simulink subsystem "PSC_AccelPdl"  (R2023a)
settings: Solver=VariableStepAuto  StartTime=0.0  StopTime=10.0  RelTol=1e-3
undefined symbols (not defined in the file or in its folder): TqCmd_Final_Forward, TqCmd_Final_Reverse
undefined symbols (not defined in the file): CAN2, ETRS, Tx
libraries: simulink x2
settings Model: Creator=edward9  LastModifiedBy=tstic

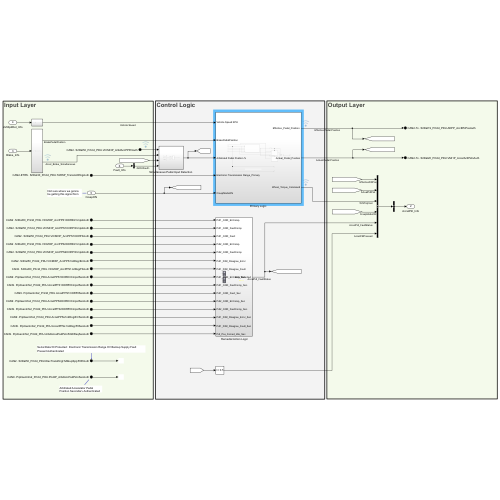
[thumbnail: Simulink's stored preview of the top-level diagram]
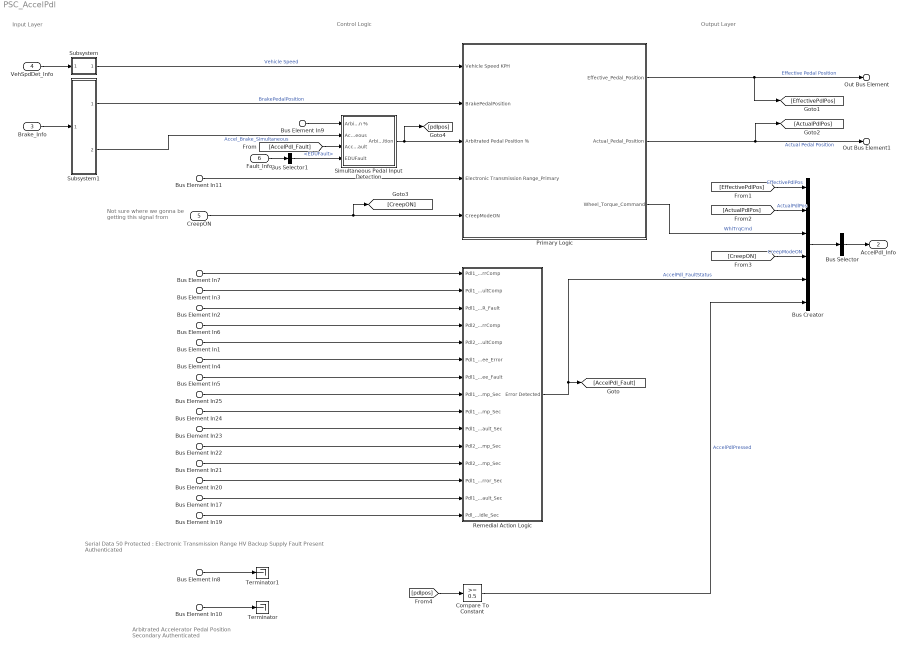
== system PSC_AccelPdl ==
  note: Output Layer
  note: Control Logic
  note: Input Layer
  note: Not sure where we gonna be getting this signal from
  note: Arbitrated Accelerator Pedal Position Secondary Authenticated
  note: Serial Data 50 Protected : Electronic Transmission Range HV Backup Supply Fault Present Authenticated
  Bus Element In7 : Inport  PortName=CAN2  Element=ID102_SrlDat50_Prtctd_PDU.VICMI3P_AccPPS1OORErrCmpstAuth
  Bus Element In3 : Inport  PortName=CAN2  Element=ID102_SrlDat50_Prtctd_PDU.VICMI3P_AccPPS1OORFltCmpstAuth
  Bus Element In2 : Inport  PortName=CAN2  Element=ID102_SrlDat50_Prtctd_PDU.VICMI3P_AccPPS1OORFltAuth
  Bus Element In6 : Inport  PortName=CAN2  Element=ID102_SrlDat50_Prtctd_PDU.VICMI3P_AccPPS2OORErrCmpstAuth
  Bus Element In1 : Inport  PortName=CAN2  Element=ID102_SrlDat50_Prtctd_PDU.VICMI3P_AccPPS2OORFltCmpstAuth
  Bus Element In4 : Inport  PortName=CAN2  Element=ID102_SrlDat50_Prtctd_PDU.VICMI3P_AccPPS1n2DsgrErrAuth
  Bus Element In5 : Inport  PortName=CAN2  Element=ID102_SrlDat50_Prtctd_PDU.VICMI3P_AccPPS1n2DsgrFltAuth
  Bus Element In8 : Inport  PortName=CAN2  Element=ID102_SrlDat50_Prtctd_PDU.ElecTransRngHVBkupSplyFltPrAuth
  Bus Element In9 : Inport  PortName=CAN2  Element=ID102_SrlDat50_Prtctd_PDU.VICMI3P_ArbdAccPPPriAuth
  Bus Element In10 : Inport  Port=2  PortName=CAN9  Element=ID106_PrplGenInfo2_Prtctd_PDU.PGI2P_ArbdAccPedPstnSecAuth
  Bus Element In25 : Inport  Port=2  PortName=CAN9  Element=ID106_PrplGenInfo2_Prtctd_PDU.AccelPPS1OORErrCmpstSecAuth
  Bus Element In24 : Inport  Port=2  PortName=CAN9  Element=ID106_PrplGenInfo2_Prtctd_PDU.AccelPPS1OORFltCmpstSecAuth
  Bus Element In23 : Inport  Port=2  PortName=CAN9  Element=ID106_PrplGenInfo2_Prtctd_PDU.AccelPPS1OORFltSecAuth
  Bus Element In22 : Inport  Port=2  PortName=CAN9  Element=ID106_PrplGenInfo2_Prtctd_PDU.AccelPPS2OORErrCmpstSecAuth
  Bus Element In21 : Inport  Port=2  PortName=CAN9  Element=ID106_PrplGenInfo2_Prtctd_PDU.AccelPPS2OORFltCmpstSecAuth
  Bus Element In20 : Inport  Port=2  PortName=CAN9  Element=ID106_PrplGenInfo2_Prtctd_PDU.AccelPPSs1n2DsgrErrSecAuth
  Bus Element In17 : Inport  Port=2  PortName=CAN9  Element=ID106_PrplGenInfo2_Prtctd_PDU.AccelPPSs1n2DsgrFltSecAuth
  Bus Element In19 : Inport  Port=2  PortName=CAN9  Element=ID106_PrplGenInfo2_Prtctd_PDU.ArbdAccelPedPstnFdIdlReqSecAuth
  Brake_Info : Inport  Port=3
  VehSpdDet_Info : Inport  Port=4
  CreepON : Inport  Port=5
  Fault_Info : Inport  Port=6
  Bus Element In11 : Inport  Port=7  PortName=CAN2-ETRS  Element=SrlDat30_Prtctd_PDU.TARSP_TransActlRngAuth
  " Remedial Action Logic" : Subsystem
  Bus Creator : BusCreator  Inputs=6
  Bus Selector : BusSelector  OutputSignals=EffectivePdlPos,ActualPdlPos,WhlTrqCmd,CreepModeON,AccelPdl_FaultStatus,AccelPdlPressed  OutputAsBus=on
  Bus Selector1 : BusSelector  OutputSignals=EDUFault
  Compare To Constant : simulink/Logic and Bit Operations/Compare To Constant  relop=>=  const=0.5  OutDataTypeStr=boolean
  "Primary Logic " : Subsystem
  "Simultaneous Pedal Input Detection " : Subsystem
  Subsystem : Subsystem
  Subsystem1 : Subsystem
  Terminator : Terminator
  Terminator1 : Terminator
  Out Bus Element : Outport  PortName=CAN2-Tx  Element=SrlDat19_Prtctd_PDU.AEPP_AccEffcPosAuth
  Out Bus Element1 : Outport  PortName=CAN2-Tx  Element=SrlDat20_Prtctd_PDU.VMI1P_AccelActlPstnAuth
  AccelPdl_Info : Outport  Port=2
  wires:
  Bus Element In11/1 -> "Primary Logic "/4(Electronic Transmission Range_Primary)
  " Remedial Action Logic"/1("Error Detected ") -> [AccelPdl_Fault], Bus Creator/5  "AccelPdl_FaultStatus"
  "Primary Logic "/3(Wheel_Torque_Command) -> Bus Creator/3  "WhlTrqCmd"
  "Primary Logic "/2(Actual_Pedal_Position) -> Out Bus Element1/1, [ActualPdlPos]  "Actual Pedal Position"
  "Primary Logic "/1("Effective_Pedal_Position ") -> Out Bus Element/1, [EffectivePdlPos]  "Effective Pedal Position"
  Bus Element In7/1 -> " Remedial Action Logic"/1(Pdl1_OOR_ErrComp)
  Bus Element In3/1 -> " Remedial Action Logic"/2(Pdl1_OOR_FaultComp)
  Bus Element In2/1 -> " Remedial Action Logic"/3(Pdl1_OOR_Fault)
  Bus Element In6/1 -> " Remedial Action Logic"/4(Pdl2_OOR_ErrComp)
  Bus Element In1/1 -> " Remedial Action Logic"/5(Pdl2_OOR_FaultComp)
  Bus Element In4/1 -> " Remedial Action Logic"/6(Pdl1_Pdl2_Disagree_Error)
  Bus Element In5/1 -> " Remedial Action Logic"/7(Pdl1_Pdl2_Disagree_Fault)
  "Simultaneous Pedal Input Detection "/1(Arbitrated Pedal Position) -> "Primary Logic "/3("Arbitrated Pedal Position % "), [pdlpos]
  Bus Element In25/1 -> " Remedial Action Logic"/8(Pdl1_OOR_ErrComp_Sec)
  Bus Element In24/1 -> " Remedial Action Logic"/9(Pdl1_OOR_FaultComp_Sec)
  Bus Element In23/1 -> " Remedial Action Logic"/10(Pdl1_OOR_Fault_Sec)
  Bus Element In22/1 -> " Remedial Action Logic"/11(Pdl2_OOR_ErrComp_Sec)
  Bus Element In21/1 -> " Remedial Action Logic"/12(Pdl2_OOR_FaultComp_Sec)
  Bus Element In20/1 -> " Remedial Action Logic"/13(Pdl1_Pdl2_Disagree_Error_Sec)
  Bus Element In17/1 -> " Remedial Action Logic"/14(Pdl1_Pdl2_Disagree_Fault_Sec)
  Bus Element In19/1 -> " Remedial Action Logic"/15(Pdl_Pos_Forced_Idle_Sec)
  CreepON/1 -> "Primary Logic "/5(CreepModeON), [CreepON]
  Bus Element In10/1 -> Terminator/1
  Bus Element In8/1 -> Terminator1/1
  VehSpdDet_Info/1 -> Subsystem/1(In1)
  Subsystem/1(VehSpd) -> "Primary Logic "/1(Vehicle Speed KPH)  "Vehicle Speed"
  Brake_Info/1 -> Subsystem1/1(Brake_Info)
  Subsystem1/1(BrakePedalPosition) -> "Primary Logic "/2(BrakePedalPosition)  "BrakePedalPosition"
  Subsystem1/2(Accel_Brake_Simultaneous) -> "Simultaneous Pedal Input Detection "/2(Accel_Brake_Simultaneous)  "Accel_Brake_Simultaneous"
  Bus Element In9/1 -> "Simultaneous Pedal Input Detection "/1("Arbitrated Pedal Position % ")
  Bus Creator/1 -> Bus Selector/1
  Bus Selector/1 -> AccelPdl_Info/1
  [AccelPdl_Fault] -> "Simultaneous Pedal Input Detection "/3(AccelPdl_Fault)
  [EffectivePdlPos] -> Bus Creator/1  "EffectivePdlPos"
  [ActualPdlPos] -> Bus Creator/2  "ActualPdlPos"
  [CreepON] -> Bus Creator/4  "CreepModeON"
  [pdlpos] -> Compare To Constant/1
  Compare To Constant/1 -> Bus Creator/6  "AccelPdlPressed"
  Fault_Info/1 -> Bus Selector1/1
  Bus Selector1/1 -> "Simultaneous Pedal Input Detection "/4(EDUFault)  "<EDUFault>"

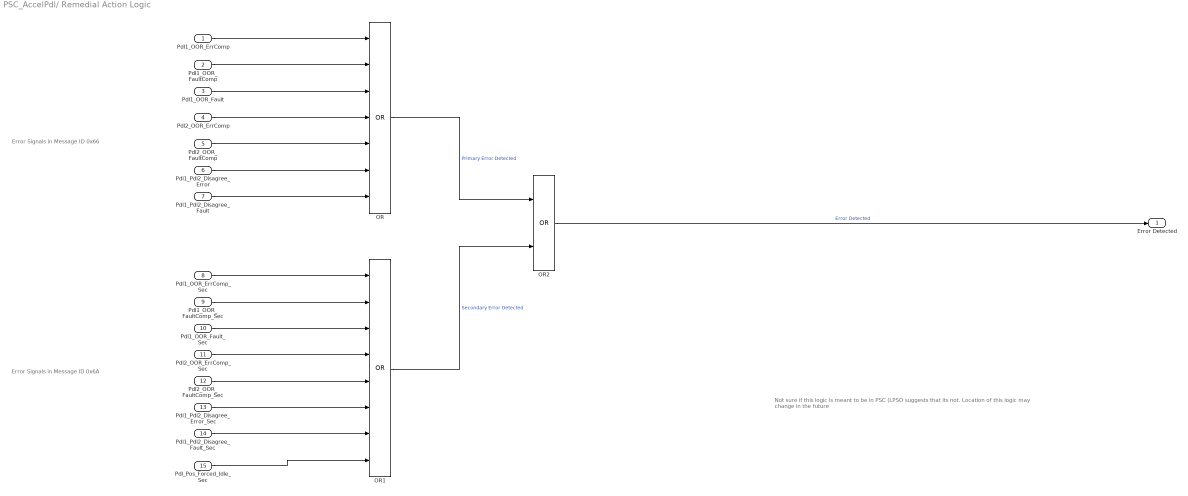
== system PSC_AccelPdl/ Remedial Action Logic ==
  note: Error Signals in Message ID 0x6A
  note: Error Signals in Message ID 0x66
  note: Not sure if this logic is meant to be in PSC (LPSO suggests that its not. Location of this logic may change in the future
  Pdl1_OOR_ErrComp : Inport
  Pdl1_OOR_FaultComp : Inport  Port=2
  Pdl1_OOR_Fault : Inport  Port=3
  Pdl2_OOR_ErrComp : Inport  Port=4
  Pdl2_OOR_FaultComp : Inport  Port=5
  Pdl1_Pdl2_Disagree_Error : Inport  Port=6
  Pdl1_Pdl2_Disagree_Fault : Inport  Port=7
  Pdl1_OOR_ErrComp_Sec : Inport  Port=8
  Pdl1_OOR_FaultComp_Sec : Inport  Port=9
  Pdl1_OOR_Fault_Sec : Inport  Port=10
  Pdl2_OOR_ErrComp_Sec : Inport  Port=11
  Pdl2_OOR_FaultComp_Sec : Inport  Port=12
  Pdl1_Pdl2_Disagree_Error_Sec : Inport  Port=13
  Pdl1_Pdl2_Disagree_Fault_Sec : Inport  Port=14
  Pdl_Pos_Forced_Idle_Sec : Inport  Port=15
  OR : Logic  Operator=OR  Inputs=7  AllPortsSameDT=off  OutDataTypeStr=boolean
  OR1 : Logic  Operator=OR  Inputs=8  AllPortsSameDT=off  OutDataTypeStr=boolean
  OR2 : Logic  Operator=OR  AllPortsSameDT=off  OutDataTypeStr=boolean
  "Error Detected " : Outport
  wires:
  Pdl_Pos_Forced_Idle_Sec/1 -> OR1/8
  OR2/1 -> "Error Detected "/1  "Error Detected"
  Pdl1_OOR_ErrComp_Sec/1 -> OR1/1
  Pdl1_OOR_Fault_Sec/1 -> OR1/3
  Pdl1_OOR_FaultComp_Sec/1 -> OR1/2
  Pdl2_OOR_ErrComp_Sec/1 -> OR1/4
  OR1/1 -> OR2/2  "Secondary Error Detected"
  Pdl2_OOR_FaultComp_Sec/1 -> OR1/5
  Pdl1_Pdl2_Disagree_Error_Sec/1 -> OR1/6
  Pdl1_Pdl2_Disagree_Fault_Sec/1 -> OR1/7
  OR/1 -> OR2/1  "Primary Error Detected"
  Pdl1_OOR_ErrComp/1 -> OR/1
  Pdl1_OOR_FaultComp/1 -> OR/2
  Pdl1_OOR_Fault/1 -> OR/3
  Pdl2_OOR_ErrComp/1 -> OR/4
  Pdl2_OOR_FaultComp/1 -> OR/5
  Pdl1_Pdl2_Disagree_Error/1 -> OR/6
  Pdl1_Pdl2_Disagree_Fault/1 -> OR/7

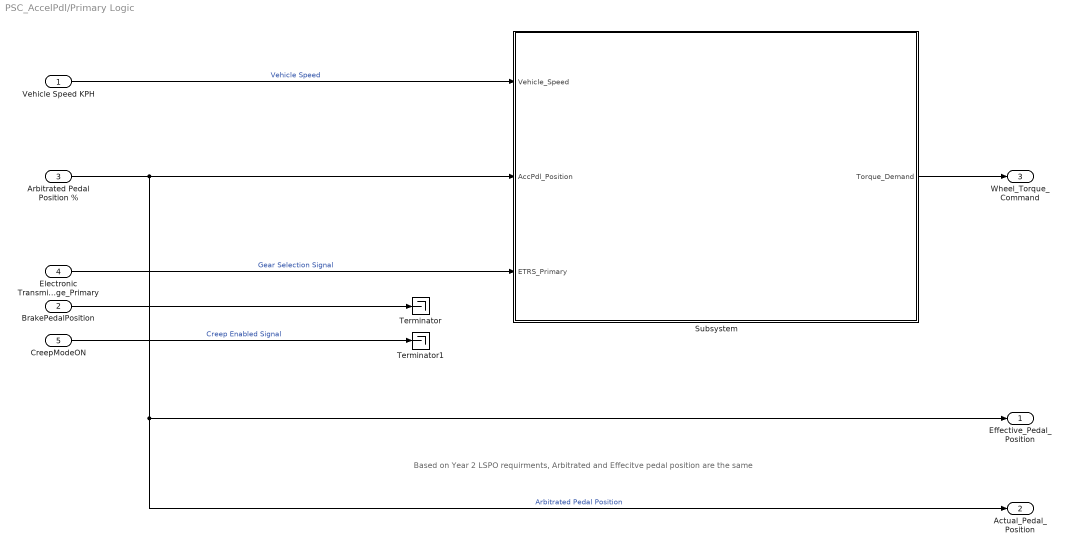
== system PSC_AccelPdl/Primary Logic  ==
  note: Based on Year 2 LSPO requirments, Arbitrated and Effecitve pedal position are the same
  Vehicle Speed KPH : Inport
  BrakePedalPosition : Inport  Port=2
  "Arbitrated Pedal Position % " : Inport  Port=3
  Electronic Transmission Range_Primary : Inport  Port=4
  CreepModeON : Inport  Port=5
  Subsystem : Subsystem
  Terminator : Terminator
  Terminator1 : Terminator
  "Effective_Pedal_Position " : Outport
  Actual_Pedal_Position : Outport  Port=2
  Wheel_Torque_Command : Outport  Port=3
  wires:
  Subsystem/1("Torque_Demand ") -> Wheel_Torque_Command/1
  BrakePedalPosition/1 -> Terminator/1
  CreepModeON/1 -> Terminator1/1  "Creep Enabled Signal"
  Electronic Transmission Range_Primary/1 -> Subsystem/3(ETRS_Primary)  "Gear Selection Signal"
  "Arbitrated Pedal Position % "/1 -> Actual_Pedal_Position/1, "Effective_Pedal_Position "/1, Subsystem/2(AccPdl_Position)  "Arbitrated Pedal Position"
  Vehicle Speed KPH/1 -> Subsystem/1(Vehicle_Speed)  "Vehicle Speed"

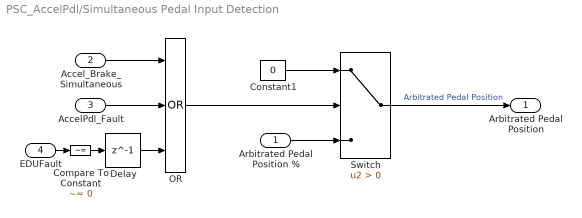
== system PSC_AccelPdl/Simultaneous Pedal Input Detection  ==
  "Arbitrated Pedal Position % " : Inport
  Accel_Brake_Simultaneous : Inport  Port=2
  AccelPdl_Fault : Inport  Port=3
  EDUFault : Inport  Port=4
  Compare To Constant : simulink/Logic and Bit Operations/Compare To Constant  relop=~=  const=0  OutDataTypeStr=boolean
  Constant1 : Constant  Value=0
  Delay : Delay  DelayLength=1
  OR : Logic  Operator=OR  Inputs=3  AllPortsSameDT=off  OutDataTypeStr=boolean
  Switch : Switch  Criteria=u2 > Threshold  SaturateOnIntegerOverflow=off  InputSameDT=off
  Arbitrated Pedal Position : Outport
  wires:
  Delay/1 -> OR/3
  Compare To Constant/1 -> Delay/1
  EDUFault/1 -> Compare To Constant/1
  AccelPdl_Fault/1 -> OR/2
  OR/1 -> Switch/2
  Switch/1 -> Arbitrated Pedal Position/1  "Arbitrated Pedal Position"
  "Arbitrated Pedal Position % "/1 -> Switch/3
  Constant1/1 -> Switch/1
  Accel_Brake_Simultaneous/1 -> OR/1

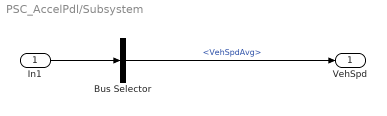
== system PSC_AccelPdl/Subsystem ==
  In1 : Inport
  Bus Selector : BusSelector  OutputSignals=VehSpdAvg
  VehSpd : Outport
  wires:
  Bus Selector/1 -> VehSpd/1  "<VehSpdAvg>"
  In1/1 -> Bus Selector/1

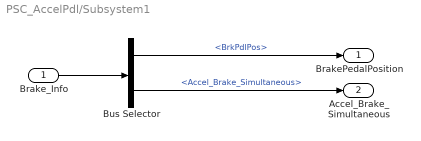
== system PSC_AccelPdl/Subsystem1 ==
  Brake_Info : Inport
  Bus Selector : BusSelector  OutputSignals=BrkPdlPos,Accel_Brake_Simultaneous
  BrakePedalPosition : Outport
  Accel_Brake_Simultaneous : Outport  Port=2
  wires:
  Bus Selector/2 -> Accel_Brake_Simultaneous/1  "<Accel_Brake_Simultaneous>"
  Bus Selector/1 -> BrakePedalPosition/1  "<BrkPdlPos>"
  Brake_Info/1 -> Bus Selector/1

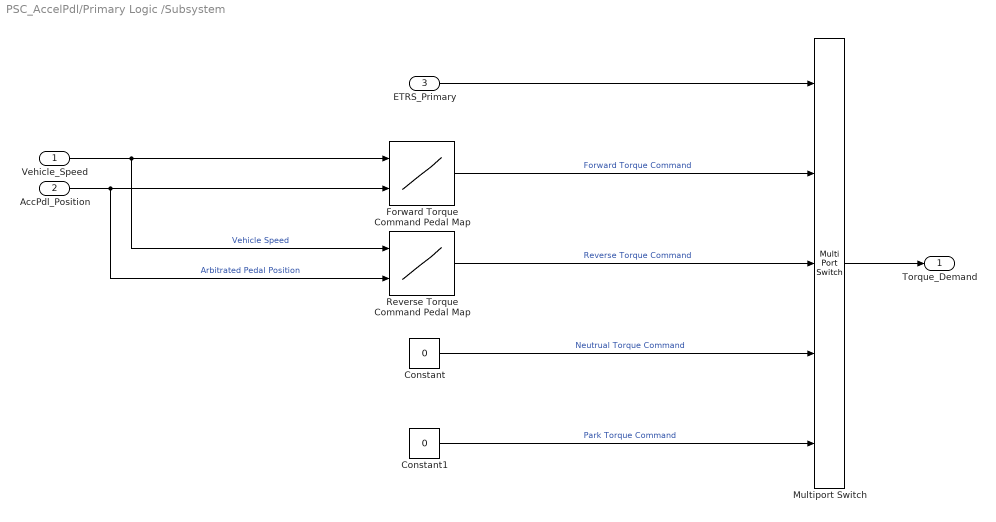
== system PSC_AccelPdl/Primary Logic /Subsystem ==
  Vehicle_Speed : Inport
  AccPdl_Position : Inport  Port=2
  ETRS_Primary : Inport  Port=3
  Constant : Constant  Value=0  SampleTime=-1
  Constant1 : Constant  Value=0  SampleTime=-1
  Forward Torque Command Pedal Map : Lookup_n-D  BreakpointsForDimension1=[0:150]  BreakpointsForDimension2=[1:100]  Table=TqCmd_Final_Forward*0.7  ExtrapMethod=Clip  UseLastTableValue=on  InternalRulePriority=Speed  RndMeth=Simplest
      settings: InputPortMap=u0,u1
  Multiport Switch : MultiPortSwitch  DataPortOrder=Specify indices  Inputs=4  DataPortIndices={7,3,5,1}  SaturateOnIntegerOverflow=off  InputSameDT=off
  Reverse Torque Command Pedal Map : Lookup_n-D  BreakpointsForDimension1=[0:150]  BreakpointsForDimension2=[1:100]  Table=TqCmd_Final_Reverse*0.15  ExtrapMethod=Clip  UseLastTableValue=on  InternalRulePriority=Speed  RndMeth=Simplest
      settings: InputPortMap=u0,u1
  "Torque_Demand " : Outport
  wires:
  Constant1/1 -> Multiport Switch/5  "Park Torque Command"
  ETRS_Primary/1 -> Multiport Switch/1
  Constant/1 -> Multiport Switch/4  "Neutrual Torque Command"
  Forward Torque Command Pedal Map/1 -> Multiport Switch/2  "Forward Torque Command"
  Multiport Switch/1 -> "Torque_Demand "/1
  Vehicle_Speed/1 -> Reverse Torque Command Pedal Map/1, Forward Torque Command Pedal Map/1  "Vehicle Speed"
  AccPdl_Position/1 -> Reverse Torque Command Pedal Map/2, Forward Torque Command Pedal Map/2  "Arbitrated Pedal Position"
  Reverse Torque Command Pedal Map/1 -> Multiport Switch/3  "Reverse Torque Command"
